simulink model "exo7self"  (R2023a)
settings: Solver=VariableStepAuto  StartTime=0.0  StopTime=10.0  RelTol=1e-3
libraries: cstblocks x4
settings Model: Creator=haoyuan  LastModifiedBy=haoyuan

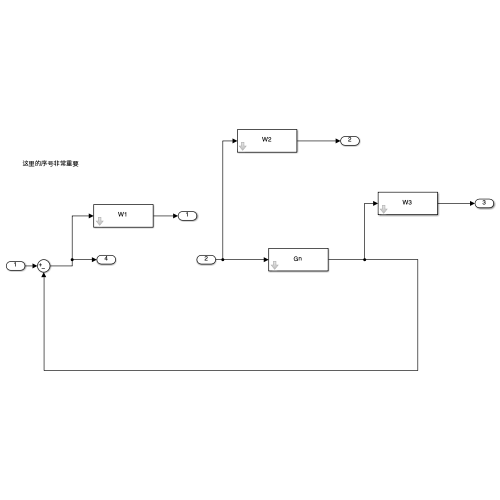
[thumbnail: Simulink's stored preview of the top-level diagram]
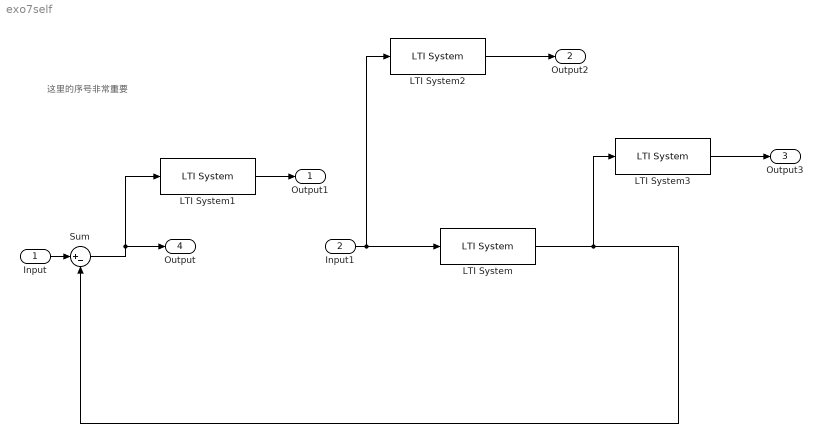
== system exo7self ==
  note: 这里的序号非常重要
  Input : Inport
  Input1 : Inport  Port=2
  LTI System : cstblocks/LTI System  sys=Gn  IC=[]
  LTI System1 : cstblocks/LTI System  sys=W1  IC=[]
  LTI System2 : cstblocks/LTI System  sys=W2  IC=[]
  LTI System3 : cstblocks/LTI System  sys=W3  IC=[]
  Sum : Sum  Inputs=|+-
  Output1 : Outport
  Output2 : Outport  Port=2
  Output3 : Outport  Port=3
  Output : Outport  Port=4
  wires:
  Input/1 -> Sum/1
  Sum/1 -> LTI System1/1, Output/1
  LTI System1/1 -> Output1/1
  LTI System/1 -> LTI System3/1, Sum/2
  Input1/1 -> LTI System/1, LTI System2/1
  LTI System2/1 -> Output2/1
  LTI System3/1 -> Output3/1
